simulink model "model"  (R2023b)
settings: Solver=VariableStepAuto  StartTime=0.0  StopTime=200  RelTol=1e-3
libraries: fuzblock x1
settings Model: Creator=chico  LastModifiedBy=diogo
settings SolverCC: AlgebraicLoopSolver=TrustRegion
settings DebuggingCC: UnconnectedInputMsg=warning  UnconnectedOutputMsg=warning  UnconnectedLineMsg=warning
settings ModelReferenceCC: EnableRefExpFcnMdlSchedulingChecks=on
settings RTWCC: DLArmComputeVersion=19.05

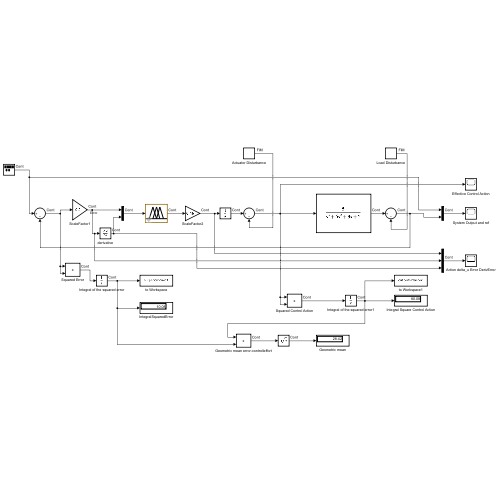
[thumbnail: Simulink's stored preview of the top-level diagram]
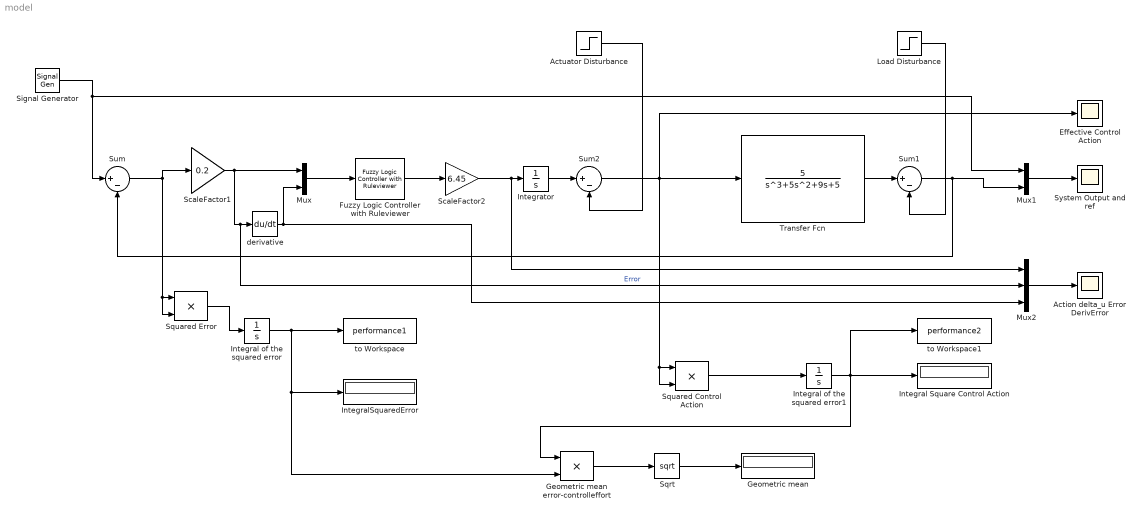
== system model ==
  Action delta_u Error DerivError : Scope
  Actuator Disturbance : Step  Time=75  SampleTime=0
  Effective Control Action : Scope
  Fuzzy Logic Controller with Ruleviewer : fuzblock/Fuzzy Logic  Controller  with Ruleviewer  fismatrix=mamdani_trimf_49r  Ts=2
  Geometric mean : Display
  Geometric mean error-controlleffort : Product
  Integral Square Control Action : Display
  Integral of the squared error : Integrator
  Integral of the squared error1 : Integrator
  IntegralSquaredError : Display
  Integrator : Integrator
  Load Disturbance : Step  Time=150  SampleTime=0
  Mux : Mux  Inputs=2
  Mux1 : Mux  Inputs=2
  Mux2 : Mux  Inputs=3
  ScaleFactor1 : Gain  Gain=0.2
  ScaleFactor2 : Gain  Gain=6.45
  Signal Generator : SignalGenerator  WaveForm=sawtooth  Frequency=0.06  Units=rad/sec
  Sqrt : Sqrt
  Squared Control Action : Product
  Squared Error : Product
  Sum : Sum  Inputs=|+-
  Sum1 : Sum  Inputs=|+-
  Sum2 : Sum  Inputs=|+-
  System Output and ref : Scope
  Transfer Fcn : TransferFcn  Numerator=[5]  Denominator=[1 5 9 5]
  derivative : Derivative
  to Workspace : ToWorkspace  VariableName=performance1  SaveFormat=Timeseries  SampleTime=-1
  to Workspace1 : ToWorkspace  VariableName=performance2  SaveFormat=Timeseries  SampleTime=-1
  wires:
  Sum/1 -> Squared Error/2, Squared Error/1, ScaleFactor1/1
  Signal Generator/1 -> Sum/1, Mux1/1
  ScaleFactor1/1 -> Mux2/2, derivative/1, Mux/1  "Error"
  derivative/1 -> Mux/2, Mux2/3
  Fuzzy Logic Controller with Ruleviewer/1 -> ScaleFactor2/1
  ScaleFactor2/1 -> Mux2/1, Integrator/1
  Integrator/1 -> Sum2/1
  Sum2/1 -> Squared Control Action/2, Squared Control Action/1, Transfer Fcn/1, Effective Control Action/1
  Actuator Disturbance/1 -> Sum2/2
  Load Disturbance/1 -> Sum1/2
  Mux1/1 -> System Output and ref/1
  Sum1/1 -> Mux1/2, Sum/2
  Mux2/1 -> Action delta_u Error DerivError/1
  Squared Error/1 -> Integral of the squared error/1
  Integral of the squared error/1 -> Geometric mean error-controlleffort/2, IntegralSquaredError/1, to Workspace/1
  Mux/1 -> Fuzzy Logic Controller with Ruleviewer/1
  Transfer Fcn/1 -> Sum1/1
  Squared Control Action/1 -> Integral of the squared error1/1
  Integral of the squared error1/1 -> Geometric mean error-controlleffort/1, to Workspace1/1, Integral Square Control Action/1
  Geometric mean error-controlleffort/1 -> Sqrt/1
  Sqrt/1 -> Geometric mean/1
